simulink model "Modelo_LTI_Equivalente"  (R2023b)
settings: Solver=VariableStepAuto  StartTime=0.0  StopTime=2  MaxStep=1e-3  RelTol=1e-3
values from neighbouring files (symbols this model uses):
  b_eq = b_m + b_l/(r^2)    (= 2.40277777778e-05)    [definicion_cte.m]
  C_ts = 0.818    [definicion_cte.m]
  J_eq = J_m + J_l/(r^2)    (= 4.58263888889e-05)    [definicion_cte.m]
  L_d = 6.6e-3    (= 0.0066)    [definicion_cte.m]
  L_ls = 0.8e-3    (= 0.0008)    [definicion_cte.m]
  L_q = 5.8e-3    (= 0.0058)    [definicion_cte.m]
  lambda_m = 0.016    [definicion_cte.m]
  P_p = 3    [definicion_cte.m]
  r = 120    [definicion_cte.m]
  R_sREF = 1.02    [definicion_cte.m]
  R_tsamb = 146.7    [definicion_cte.m]
  T_amb = 25    [definicion_cte.m]
libraries: SignalEditorBlockLib x2
settings Model: Creator=MSI  LastModifiedBy=MSI

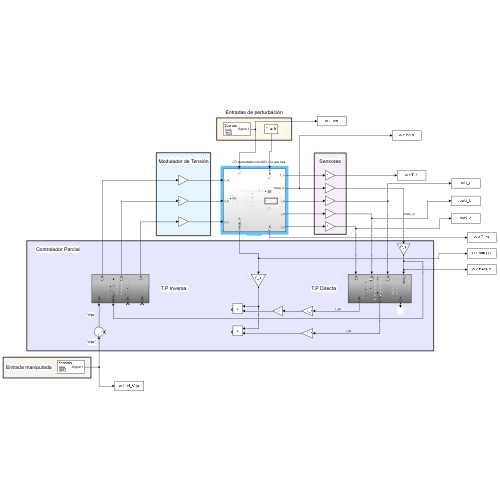
[thumbnail: Simulink's stored preview of the top-level diagram]
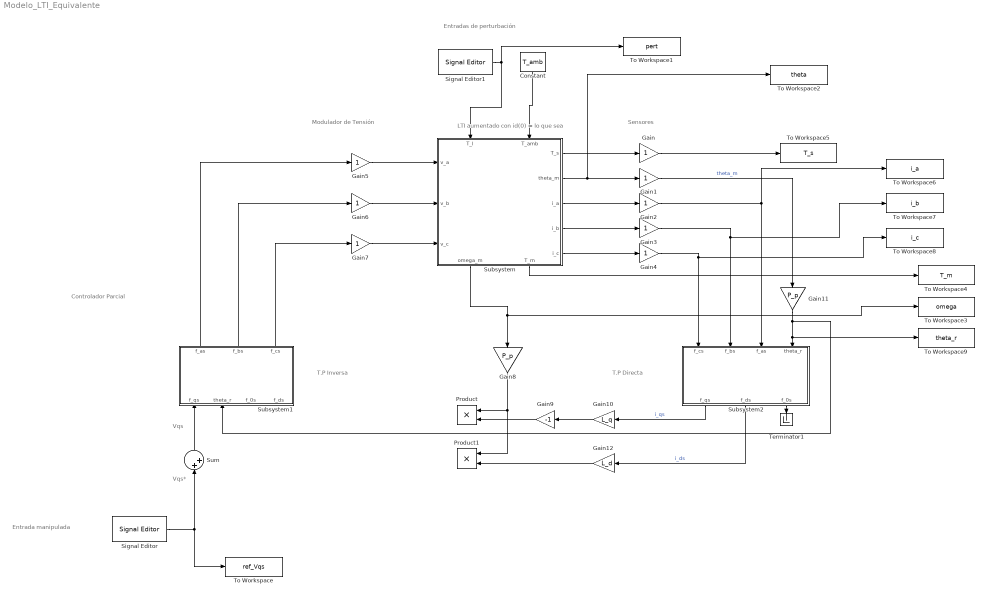
== system Modelo_LTI_Equivalente ==
  note: Vqs
  note: Sensores
  note: T.P Directa
  note: T.P Inversa
  note: LTI aumentado con id(0) = lo que sea
  note: Entradas de perturbación
  note: Entrada manipulada
  note: Vqs*
  note: Modulador de Tensión
  note: Controlador Parcial
  Constant : Constant  Value=T_amb
  Gain{,1..7} (8 alike) : Gain
  Gain10 : Gain  Gain=L_q
  Gain11 : Gain  Gain=P_p
  Gain12 : Gain  Gain=L_d
  Gain8 : Gain  Gain=P_p
  Gain9 : Gain  Gain=-1
  Product : Product
  Product1 : Product
  Signal Editor : SignalEditorBlockLib/Signal Editor  FileName=Vq.mat  ActiveScenario=Scenario  ActiveSignal=Signal 1  IsBus=off  OutputBusObjectStr=Bus: BusObject  SampleTime=0  Interpolate=off  ZeroCross=off  OutputAfterFinalValue=Setting to zero  Unit=inherit  PreserveSignalName=on  ApplySigPropsToAllScenarios=on  ApplySigPropsToAllSignals=off
  Signal Editor1 : SignalEditorBlockLib/Signal Editor  FileName=C:\Users\MSI\Documents\FING\Materias\AyME\Repo_proyecto\AyME\Avances_Sito\Tl.mat  ActiveScenario=Scenario  ActiveSignal=Signal 1  IsBus=off  OutputBusObjectStr=Bus: BusObject  SampleTime=0  Interpolate=off  ZeroCross=off  OutputAfterFinalValue=Setting to zero  Unit=inherit  PreserveSignalName=on  ApplySigPropsToAllScenarios=on  ApplySigPropsToAllSignals=off
  Subsystem : Subsystem
      settings: PortSchema="{\"entries\":[{\"content\":{\"sides\":[{\"content\":{\"connectorIds\":[\"In1\",\"In2\",\"In3\"]},\"type\":\"ConnectorPlacement.EquallySpacedRectSide\",\"uuid\":\"bb514e72-0884-4524-a507-3a7e4e273755\"},{\"content\":{\"connectorIds\":[\"Out1\",\"Out2\",\"Out3\",\"Out4\",\"Out5\"],\"side\":\"RIGHT\"},\"type\":\"ConnectorPlacement.EquallySpacedRectSide\",\"uuid\":\"481d9492-5179-49c8-92cd-b60559a6f669\"},{\"content\":{\"connectorIds\":[\"In4\",\"In5\"],\"side\":\"TOP\"},\"type\":\"ConnectorPlacement.EquallySpacedRectSide\",\"uuid\":\"6eb99a34-8af8-461b-8a76-2bbbe7c0805f\"},{\"content\":{\"connectorIds\":[\"Out6\",\"Out7\"],\"side\":\"BOTTOM\"},\"type\":\"ConnectorPlacement.EquallySpacedRectSide\",\"uuid\":\"2710cae4-50fb-43ae-b722-5b22c6c50617\"}]},\"type\":\"ConnectorPlacement.EquallySpacedConnector\",\"uuid\":\"6257ea4d-8f33-47d0-8dc0-e891171582bf\"}],\"packageUris\":[\"http://schema.mathworks.com/mf0/Connector/R2020b\"],\"version\":\"1.0\"}"
  Subsystem1 : Subsystem
  Subsystem2 : Subsystem
  Sum : Sum  Inputs=|++
  Terminator1 : Terminator
  To Workspace : ToWorkspace  VariableName=ref_Vqs  SaveFormat=Timeseries  SampleTime=-1
  To Workspace1 : ToWorkspace  VariableName=pert  SaveFormat=Timeseries  SampleTime=-1
  To Workspace2 : ToWorkspace  VariableName=theta  SaveFormat=Timeseries  SampleTime=-1
  To Workspace3 : ToWorkspace  VariableName=omega  SaveFormat=Timeseries  SampleTime=-1
  To Workspace4 : ToWorkspace  VariableName=T_m  SaveFormat=Timeseries  SampleTime=-1
  To Workspace5 : ToWorkspace  VariableName=T_s  SaveFormat=Timeseries  SampleTime=-1
  To Workspace6 : ToWorkspace  VariableName=i_a  SaveFormat=Timeseries  SampleTime=-1
  To Workspace7 : ToWorkspace  VariableName=i_b  SaveFormat=Timeseries  SampleTime=-1
  To Workspace8 : ToWorkspace  VariableName=i_c  SaveFormat=Timeseries  SampleTime=-1
  To Workspace9 : ToWorkspace  VariableName=theta_r  SaveFormat=Timeseries  SampleTime=-1
  wires:
  Subsystem/2(theta_m) -> To Workspace2/1, Gain1/1
  Subsystem/3(i_a) -> Gain2/1
  Subsystem/6(omega_m) -> To Workspace3/1, Gain8/1
  Gain2/1 -> Subsystem2/3(f_as), To Workspace6/1
  Gain7/1 -> Subsystem/3(v_c)
  Subsystem2/3(f_0s) -> Terminator1/1
  Gain12/1 -> Product1/2
  Gain10/1 -> Gain9/1
  Subsystem2/2(f_ds) -> Gain12/1  "i_ds"
  Gain4/1 -> Subsystem2/1(f_cs), To Workspace8/1
  Subsystem1/3(f_cs) -> Gain7/1
  Gain9/1 -> Product/2
  Subsystem1/2(f_bs) -> Gain6/1
  Subsystem2/1(f_qs) -> Gain10/1  "i_qs"
  Gain1/1 -> Gain11/1  "theta_m"
  Signal Editor1/1 -> Subsystem/4(T_l), To Workspace1/1
  Gain8/1 -> Product1/1, Product/1
  Subsystem1/1(f_as) -> Gain5/1
  Signal Editor/1 -> To Workspace/1, Sum/1
  Sum/1 -> Subsystem1/1(f_qs)
  Gain11/1 -> Subsystem1/2(theta_r), To Workspace9/1, Subsystem2/4(theta_r)
  Subsystem/5(i_c) -> Gain4/1
  Subsystem/1(T_s) -> Gain/1
  Gain/1 -> To Workspace5/1
  Subsystem/7(T_m) -> To Workspace4/1
  Gain5/1 -> Subsystem/1(v_a)
  Constant/1 -> Subsystem/5(T_amb)
  Gain3/1 -> To Workspace7/1, Subsystem2/2(f_bs)
  Subsystem/4(i_b) -> Gain3/1
  Gain6/1 -> Subsystem/2(v_b)

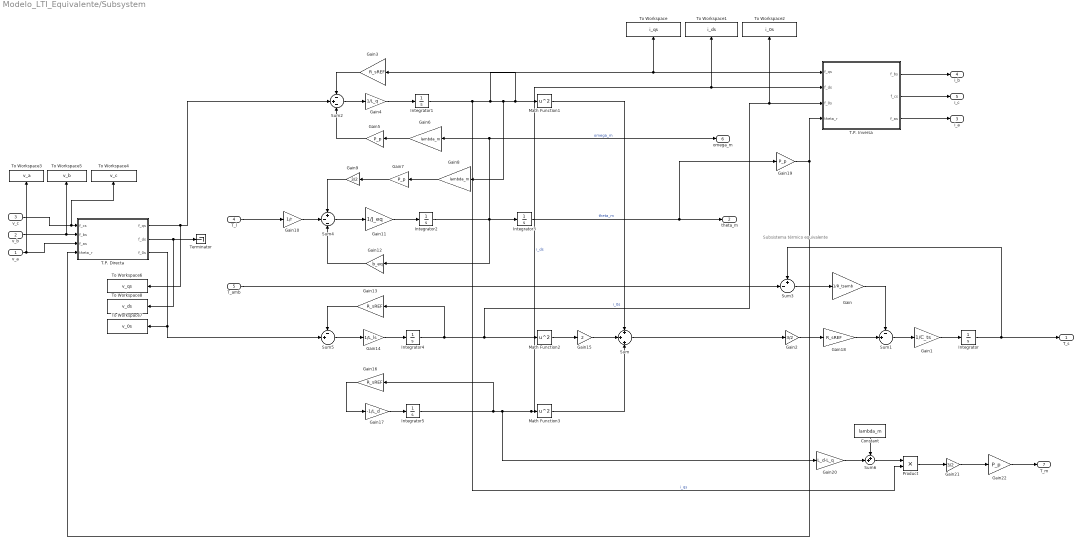
== system Modelo_LTI_Equivalente/Subsystem ==
  note: Subsistema térmico equivalente
  v_a : Inport
  v_b : Inport  Port=2
  v_c : Inport  Port=3
  T_l : Inport  Port=4
  T_amb : Inport  Port=5
  Constant : Constant  Value=lambda_m
  Gain : Gain  Gain=1/R_tsamb
  Gain1 : Gain  Gain=1/C_ts
  Gain10 : Gain  Gain=1/r
  Gain11 : Gain  Gain=1/J_eq
  Gain12 : Gain  Gain=b_eq
  Gain{3,13,16,18} (4 alike) : Gain  Gain=R_sREF
  Gain14 : Gain  Gain=1/L_ls
  Gain15 : Gain  Gain=2
  Gain17 : Gain  Gain=-1/L_d
  Gain{5,7,19,22} (4 alike) : Gain  Gain=P_p
  Gain2 : Gain  Gain=3/2
  Gain20 : Gain  Gain=L_d-L_q
  Gain21 : Gain  Gain=3/2
  Gain4 : Gain  Gain=1/L_q
  Gain6 : Gain  Gain=lambda_m
  Gain8 : Gain  Gain=lambda_m
  Gain9 : Gain  Gain=3/2
  Integrator{,1..5} (6 alike) : Integrator
  Math Function1 : Math  Operator=square
  Math Function2 : Math  Operator=square
  Math Function3 : Math  Operator=square
  Product : Product
  Sum : Sum  Inputs=+|+|+
  Sum1 : Sum  Inputs=-+|
  Sum2 : Sum  Inputs=-+-
  Sum3 : Sum  Inputs=+-|
  Sum4 : Sum  Inputs=+--
  Sum5 : Sum  Inputs=-+|
  Sum6 : Sum  Inputs=++|
  T.P. Directa : Subsystem
  T.P. Inversa : Subsystem
  Terminator : Terminator
  To Workspace : ToWorkspace  VariableName=i_qs  SaveFormat=Timeseries  SampleTime=-1
  To Workspace1 : ToWorkspace  VariableName=i_ds  SaveFormat=Timeseries  SampleTime=-1
  To Workspace2 : ToWorkspace  VariableName=i_0s  SaveFormat=Timeseries  SampleTime=-1
  To Workspace3 : ToWorkspace  VariableName=v_a  SaveFormat=Timeseries  SampleTime=-1
  To Workspace4 : ToWorkspace  VariableName=v_c  SaveFormat=Timeseries  SampleTime=-1
  To Workspace5 : ToWorkspace  VariableName=v_b  SaveFormat=Timeseries  SampleTime=-1
  To Workspace6 : ToWorkspace  VariableName=v_qs  SaveFormat=Timeseries  SampleTime=-1
  To Workspace7 : ToWorkspace  VariableName=v_0s  SaveFormat=Timeseries  SampleTime=-1
  To Workspace8 : ToWorkspace  VariableName=v_ds  SaveFormat=Timeseries  SampleTime=-1
  T_s : Outport
  theta_m : Outport  Port=2
  i_a : Outport  Port=3
  i_b : Outport  Port=4
  i_c : Outport  Port=5
  omega_m : Outport  Port=6
  T_m : Outport  Port=7
  wires:
  T.P. Inversa/3(f_as) -> i_a/1
  Integrator4/1 -> T.P. Inversa/3(f_0s), To Workspace2/1, Math Function2/1, Gain13/1  "i_0s"
  Math Function2/1 -> Gain15/1
  Integrator3/1 -> theta_m/1, Gain19/1  "theta_m"
  Integrator/1 -> T_s/1, Sum3/1
  Gain11/1 -> Integrator2/1
  Sum2/1 -> Gain4/1
  T.P. Inversa/1(f_bs) -> i_b/1
  Integrator2/1 -> Integrator3/1, Gain12/1, omega_m/1, Gain6/1  "omega_m"
  Integrator1/1 -> Product/2, To Workspace/1, T.P. Inversa/1(f_qs), Gain3/1, Math Function1/1, Gain8/1  "i_qs"
  Sum5/1 -> Gain14/1
  Gain4/1 -> Integrator1/1
  T.P. Directa/3(f_0s) -> To Workspace7/1, Sum5/2
  T.P. Inversa/2(f_cs) -> i_c/1
  T.P. Directa/1(f_qs) -> Sum2/2, To Workspace6/1
  Gain3/1 -> Sum2/1
  Gain5/1 -> Sum2/3
  Gain1/1 -> Integrator/1
  Math Function1/1 -> Sum/1
  Gain19/1 -> T.P. Inversa/4(theta_r), T.P. Directa/4(theta_r)
  Sum/1 -> Gain2/1
  Integrator5/1 -> Gain16/1, Gain20/1, To Workspace1/1, T.P. Inversa/2(f_ds), Math Function3/1  "i_ds"
  Gain10/1 -> Sum4/2
  Gain7/1 -> Gain9/1
  Gain9/1 -> Sum4/1
  Sum4/1 -> Gain11/1
  Gain12/1 -> Sum4/3
  Sum3/1 -> Gain/1
  Gain18/1 -> Sum1/2
  Gain6/1 -> Gain5/1
  Gain15/1 -> Sum/2
  Gain17/1 -> Integrator5/1
  Gain/1 -> Sum1/1
  Gain13/1 -> Sum5/1
  Math Function3/1 -> Sum/3
  Gain14/1 -> Integrator4/1
  T_amb/1 -> Sum3/2
  T_l/1 -> Gain10/1
  Gain8/1 -> Gain7/1
  Gain16/1 -> Gain17/1
  Gain2/1 -> Gain18/1
  Sum1/1 -> Gain1/1
  Gain22/1 -> T_m/1
  Sum6/1 -> Product/1
  Gain21/1 -> Gain22/1
  Constant/1 -> Sum6/1
  Gain20/1 -> Sum6/2
  Product/1 -> Gain21/1
  T.P. Directa/2(f_ds) -> To Workspace8/1, Terminator/1
  v_a/1 -> T.P. Directa/3(f_as), To Workspace3/1
  v_b/1 -> To Workspace5/1, T.P. Directa/2(f_bs)
  v_c/1 -> To Workspace4/1, T.P. Directa/1(f_cs)

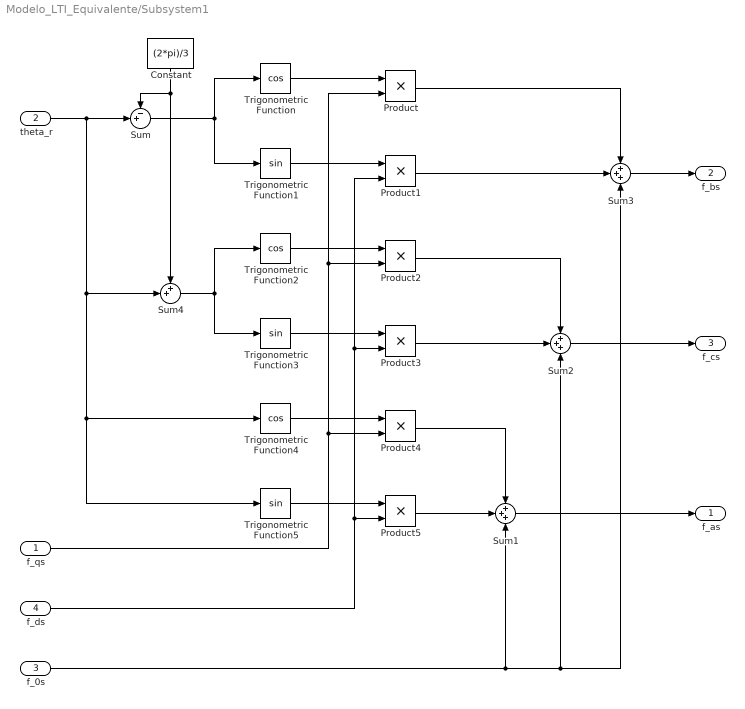
== system Modelo_LTI_Equivalente/Subsystem1 ==
  f_qs : Inport
  theta_r : Inport  Port=2
  f_0s : Inport  Port=3
  f_ds : Inport  Port=4
  Constant : Constant  Value=(2*pi)/3
  Product{,1..5} (6 alike) : Product
  Sum : Sum  Inputs=-+|
  Sum1 : Sum  Inputs=+++
  Sum2 : Sum  Inputs=+++
  Sum3 : Sum  Inputs=+++
  Sum4 : Sum  Inputs=++|
  Trigonometric Function : Trigonometry  Operator=cos
  Trigonometric Function1 : Trigonometry
  Trigonometric Function2 : Trigonometry  Operator=cos
  Trigonometric Function3 : Trigonometry
  Trigonometric Function4 : Trigonometry  Operator=cos
  Trigonometric Function5 : Trigonometry
  f_as : Outport
  f_bs : Outport  Port=2
  f_cs : Outport  Port=3
  wires:
  Sum1/1 -> f_as/1
  Product5/1 -> Sum1/2
  Sum2/1 -> f_cs/1
  Product1/1 -> Sum3/2
  Trigonometric Function5/1 -> Product5/1
  Sum/1 -> Trigonometric Function1/1, Trigonometric Function/1
  Product2/1 -> Sum2/1
  Product4/1 -> Sum1/1
  f_qs/1 -> Product4/2, Product2/2, Product/2
  Product/1 -> Sum3/1
  f_0s/1 -> Sum3/3, Sum2/3, Sum1/3
  Trigonometric Function4/1 -> Product4/1
  Constant/1 -> Sum4/1, Sum/1
  Trigonometric Function2/1 -> Product2/1
  f_ds/1 -> Product5/2, Product3/2, Product1/2
  Trigonometric Function3/1 -> Product3/1
  Trigonometric Function1/1 -> Product1/1
  Sum4/1 -> Trigonometric Function3/1, Trigonometric Function2/1
  Sum3/1 -> f_bs/1
  theta_r/1 -> Sum4/2, Trigonometric Function5/1, Trigonometric Function4/1, Sum/2
  Product3/1 -> Sum2/2
  Trigonometric Function/1 -> Product/1

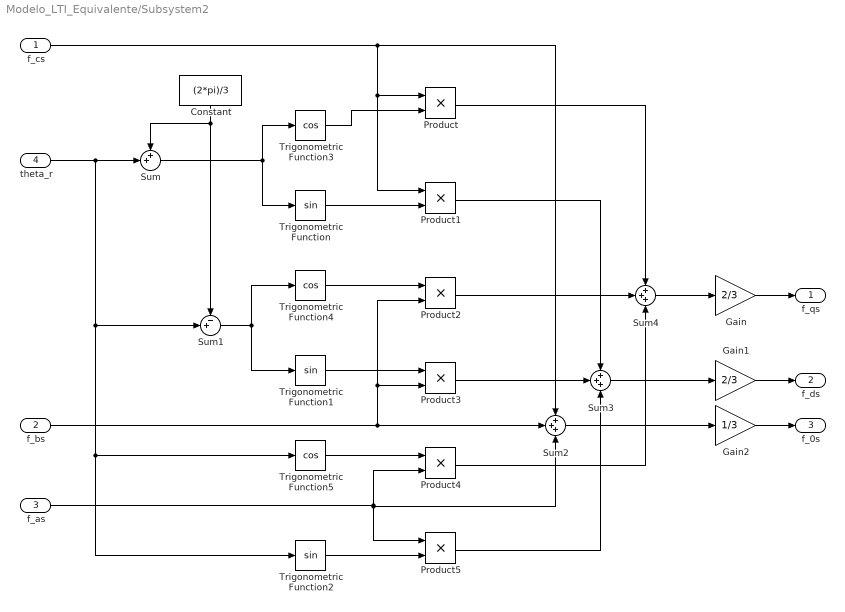
== system Modelo_LTI_Equivalente/Subsystem2 ==
  f_cs : Inport
  f_bs : Inport  Port=2
  f_as : Inport  Port=3
  theta_r : Inport  Port=4
  Constant : Constant  Value=(2*pi)/3
  Gain : Gain  Gain=2/3
  Gain1 : Gain  Gain=2/3
  Gain2 : Gain  Gain=1/3
  Product{,1..5} (6 alike) : Product
  Sum : Sum  Inputs=++|
  Sum1 : Sum  Inputs=-+|
  Sum2 : Sum  Inputs=+++
  Sum3 : Sum  Inputs=+++
  Sum4 : Sum  Inputs=+++
  Trigonometric Function : Trigonometry
  Trigonometric Function1 : Trigonometry
  Trigonometric Function2 : Trigonometry
  Trigonometric Function3 : Trigonometry  Operator=cos
  Trigonometric Function4 : Trigonometry  Operator=cos
  Trigonometric Function5 : Trigonometry  Operator=cos
  f_qs : Outport
  f_ds : Outport  Port=2
  f_0s : Outport  Port=3
  wires:
  f_cs/1 -> Product/1, Product1/1, Sum2/1
  Product3/1 -> Sum3/2
  Trigonometric Function5/1 -> Product4/1
  Constant/1 -> Sum/1, Sum1/1
  Sum1/1 -> Trigonometric Function1/1, Trigonometric Function4/1
  Gain2/1 -> f_0s/1
  Gain1/1 -> f_ds/1
  theta_r/1 -> Sum1/2, Trigonometric Function2/1, Trigonometric Function5/1, Sum/2
  Sum4/1 -> Gain/1
  Trigonometric Function1/1 -> Product3/1
  f_bs/1 -> Product2/2, Product3/2, Sum2/2
  Product4/1 -> Sum4/3
  Gain/1 -> f_qs/1
  Product/1 -> Sum4/1
  f_as/1 -> Sum2/3, Product5/1, Product4/2
  Sum2/1 -> Gain2/1
  Product2/1 -> Sum4/2
  Trigonometric Function2/1 -> Product5/2
  Sum3/1 -> Gain1/1
  Trigonometric Function/1 -> Product1/2
  Trigonometric Function3/1 -> Product/2
  Trigonometric Function4/1 -> Product2/1
  Product5/1 -> Sum3/3
  Product1/1 -> Sum3/1
  Sum/1 -> Trigonometric Function3/1, Trigonometric Function/1

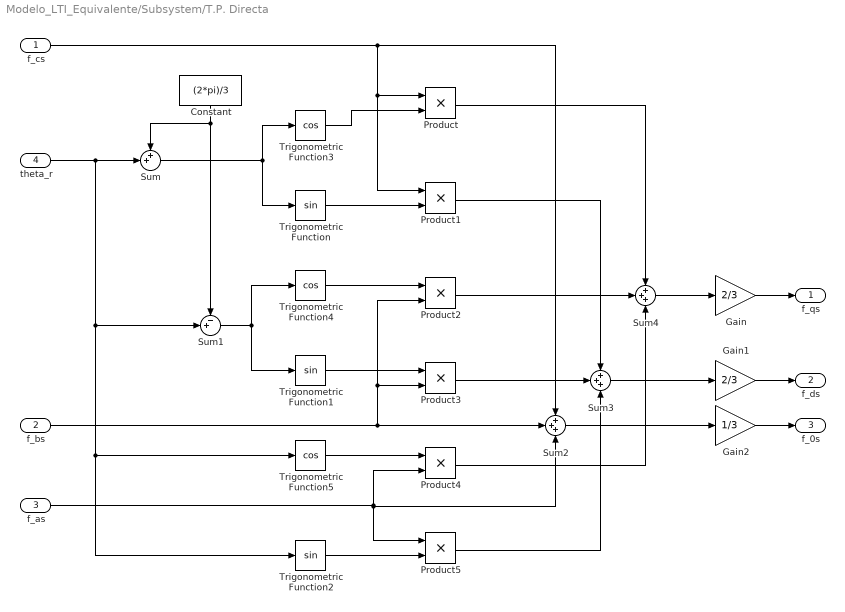
== system Modelo_LTI_Equivalente/Subsystem/T.P. Directa ==
  f_cs : Inport
  f_bs : Inport  Port=2
  f_as : Inport  Port=3
  theta_r : Inport  Port=4
  Constant : Constant  Value=(2*pi)/3
  Gain : Gain  Gain=2/3
  Gain1 : Gain  Gain=2/3
  Gain2 : Gain  Gain=1/3
  Product{,1..5} (6 alike) : Product
  Sum : Sum  Inputs=++|
  Sum1 : Sum  Inputs=-+|
  Sum2 : Sum  Inputs=+++
  Sum3 : Sum  Inputs=+++
  Sum4 : Sum  Inputs=+++
  Trigonometric Function : Trigonometry
  Trigonometric Function1 : Trigonometry
  Trigonometric Function2 : Trigonometry
  Trigonometric Function3 : Trigonometry  Operator=cos
  Trigonometric Function4 : Trigonometry  Operator=cos
  Trigonometric Function5 : Trigonometry  Operator=cos
  f_qs : Outport
  f_ds : Outport  Port=2
  f_0s : Outport  Port=3
  wires:
  Product5/1 -> Sum3/3
  theta_r/1 -> Sum1/2, Trigonometric Function2/1, Trigonometric Function5/1, Sum/2
  f_bs/1 -> Product2/2, Product3/2, Sum2/2
  f_cs/1 -> Product/1, Product1/1, Sum2/1
  Trigonometric Function5/1 -> Product4/1
  Sum1/1 -> Trigonometric Function1/1, Trigonometric Function4/1
  Constant/1 -> Sum/1, Sum1/1
  Sum/1 -> Trigonometric Function3/1, Trigonometric Function/1
  f_as/1 -> Sum2/3, Product5/1, Product4/2
  Gain2/1 -> f_0s/1
  Trigonometric Function2/1 -> Product5/2
  Trigonometric Function1/1 -> Product3/1
  Product/1 -> Sum4/1
  Sum4/1 -> Gain/1
  Trigonometric Function3/1 -> Product/2
  Gain/1 -> f_qs/1
  Gain1/1 -> f_ds/1
  Product2/1 -> Sum4/2
  Product1/1 -> Sum3/1
  Product4/1 -> Sum4/3
  Product3/1 -> Sum3/2
  Sum2/1 -> Gain2/1
  Trigonometric Function4/1 -> Product2/1
  Trigonometric Function/1 -> Product1/2
  Sum3/1 -> Gain1/1

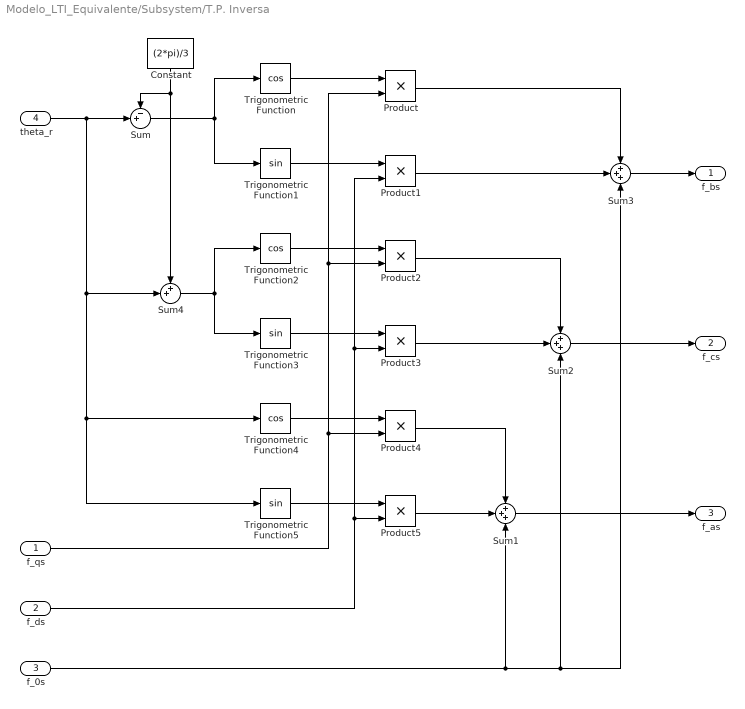
== system Modelo_LTI_Equivalente/Subsystem/T.P. Inversa ==
  f_qs : Inport
  f_ds : Inport  Port=2
  f_0s : Inport  Port=3
  theta_r : Inport  Port=4
  Constant : Constant  Value=(2*pi)/3
  Product{,1..5} (6 alike) : Product
  Sum : Sum  Inputs=-+|
  Sum1 : Sum  Inputs=+++
  Sum2 : Sum  Inputs=+++
  Sum3 : Sum  Inputs=+++
  Sum4 : Sum  Inputs=++|
  Trigonometric Function : Trigonometry  Operator=cos
  Trigonometric Function1 : Trigonometry
  Trigonometric Function2 : Trigonometry  Operator=cos
  Trigonometric Function3 : Trigonometry
  Trigonometric Function4 : Trigonometry  Operator=cos
  Trigonometric Function5 : Trigonometry
  f_bs : Outport
  f_cs : Outport  Port=2
  f_as : Outport  Port=3
  wires:
  theta_r/1 -> Sum4/2, Trigonometric Function5/1, Trigonometric Function4/1, Sum/2
  Trigonometric Function3/1 -> Product3/1
  Product4/1 -> Sum1/1
  Product1/1 -> Sum3/2
  Trigonometric Function2/1 -> Product2/1
  Product2/1 -> Sum2/1
  f_0s/1 -> Sum3/3, Sum2/3, Sum1/3
  f_qs/1 -> Product4/2, Product2/2, Product/2
  Product5/1 -> Sum1/2
  Trigonometric Function1/1 -> Product1/1
  Sum/1 -> Trigonometric Function1/1, Trigonometric Function/1
  Trigonometric Function5/1 -> Product5/1
  Sum4/1 -> Trigonometric Function3/1, Trigonometric Function2/1
  Product/1 -> Sum3/1
  Product3/1 -> Sum2/2
  Trigonometric Function/1 -> Product/1
  Sum2/1 -> f_cs/1
  Sum3/1 -> f_bs/1
  f_ds/1 -> Product5/2, Product3/2, Product1/2
  Trigonometric Function4/1 -> Product4/1
  Sum1/1 -> f_as/1
  Constant/1 -> Sum4/1, Sum/1
